simulink model "atakanproje2020a"  (R2020a)
settings: Solver=VariableStepAuto  StartTime=0.0  StopTime=5  RelTol=1e-3
libraries: powerlib x11, powerlib_meascontrol x6, simulink x4, eeAsmScalarControl x1
settings Model: Creator=Atakan  LastModifiedBy=Atakan
settings DebuggingCC: ArithmeticOperatorsInVariantConditions=warning
settings SFSimCC: CustomCodeUndefinedFunction=UseInterfaceOnly

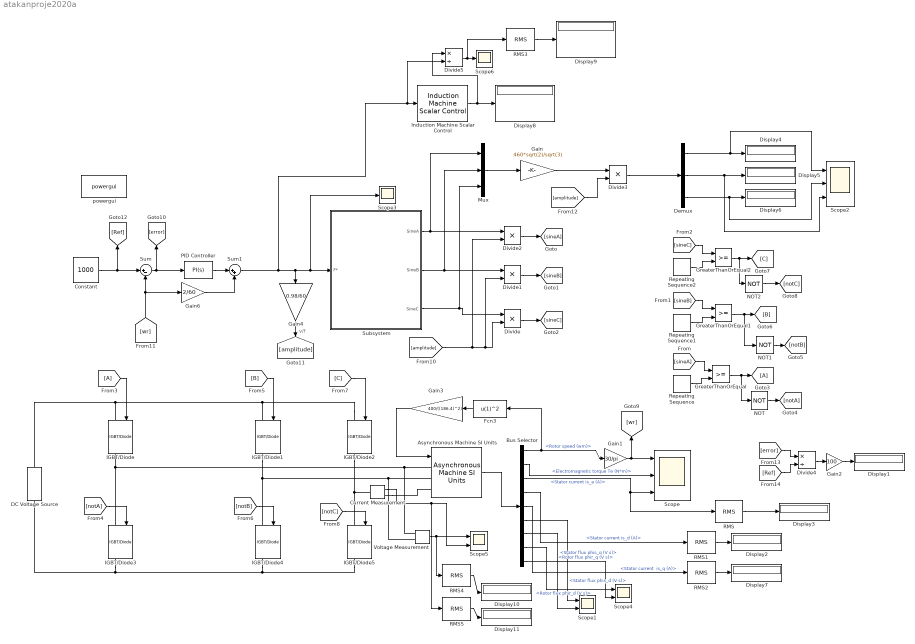
== system atakanproje2020a ==
  note: v/f
  Asynchronous Machine SI Units : powerlib/Machines/Asynchronous Machine SI Units  RotorType=Squirrel-cage  PresetModel="05:  100 HP 460 V 60Hz 1780 RPM"  MechanicalLoad=Torque Tm  ShowDetailedParameters=on  ReferenceFrame=Rotor  Units=SI  MeasurementBus=off  NominalParameters=[7.46e+04 460 60]  Stator=[0.03957 0.000389]  Rotor=[0.02215 0.000389]  Cage1=[0.4155 0.002066]  Cage2=[0.4168 0.0003495]  Lm=0.01664  Mechanical=[1.3 0.05543 2]  PolePairs=2  InitialConditions=[1 0 0 0 0 0 0 0]  SimulateSaturation=off  Saturation=[14.03593122, 27.81365428, 53.79336849, 72.68890987, 97.98006896, 148.6815601, 215.7428561, 302.9841135, 428.7778367 ; 230, 322, 414, 460, 506, 552, 598, 644, 690]  LoadFlowParameters=1492000  TsPowergui=0  TsBlock=-1  IterativeModel=Trapezoidal non iterative  IterativeDiscreteModel=Trapezoidal non iterative  Pmec=1.492e+006
  Bus Selector : BusSelector  OutputSignals="Mechanical.Rotor speed (wm),Mechanical.Electromagnetic torque Te (N*m),Stator measurements.Stator current is_a (A),Stator measurements.Stator current is_d (A),Stator measurements.Stator current  is_q (A),Stator measurements.Stator flux phis_d (V s),Stator measurements.Stator flux phis_q (V s),Rotor measurements.Rotor flux phir_d (V s),Rotor measurements.Rotor flux phir_q (V s)"
  Constant : Constant  Value=1000
  Current Measurement : powerlib/Measurements/Current Measurement  PhasorSimulation=off  OutputType=Complex  PSBequivalent=0
  DC Voltage Source : powerlib/Electrical Sources/DC Voltage Source  Amplitude=800  Measurements=None
  Demux : Demux  Outputs=3
  Display{1..11} (11 alike) : Display
  Divide{,1..3} (4 alike) : Product  Inputs=**
  Divide4 : Product  Inputs=*/
  Divide5 : Product  Inputs=*/
  Fcn3 : Fcn  Expr=u(1)^2
  Gain : Gain  Gain=460*sqrt(2)/sqrt(3)
  Gain1 : Gain  Gain=30/pi
  Gain2 : Gain  Gain=100
  Gain3 : Gain  Gain=400/((186.4)^2)
  Gain4 : Gain  Gain=0.98/60
  Gain6 : Gain  Gain=2/60
  GreaterThanOrEqual : RelationalOperator  OutDataTypeStr=boolean  RndMeth=Simplest
  GreaterThanOrEqual1 : RelationalOperator  OutDataTypeStr=boolean  RndMeth=Simplest
  GreaterThanOrEqual2 : RelationalOperator  OutDataTypeStr=boolean  RndMeth=Simplest
  IGBT/Diode{,1..5} (6 alike) : powerlib/Power Electronics/IGBT//Diode  Ron=1e-3  Rs=1e5  Cs=inf  Measurements=on
  Induction Machine Scalar Control : eeAsmScalarControl/Induction Machine Scalar Control  fn=60  Vn=460  Vmin=10  Ts=-1
      settings: SourceProductBaseCode=PS
  Mux : Mux  Inputs=3
  NOT : Logic  Operator=NOT  AllPortsSameDT=off  OutDataTypeStr=boolean
  NOT1 : Logic  Operator=NOT  AllPortsSameDT=off  OutDataTypeStr=boolean
  NOT2 : Logic  Operator=NOT  AllPortsSameDT=off  OutDataTypeStr=boolean
  PID Controller : simulink/Continuous/PID Controller  Controller=PI  Form=Parallel  TimeDomain=Continuous-time  UseExternalTs=off  SampleTime=-1  IntegratorMethod=Forward Euler  FilterMethod=Forward Euler  ControllerParametersSource=internal  P=0.01  I=0.0001  D=0.000001  UseFilter=on  N=100  TunerSelectOption=Transfer Function Based (PID Tuner App)  InitialConditionSource=internal  InitialConditionForIntegrator=0  InitialConditionForFilter=0  DifferentiatorICPrevScaledInput=0  ExternalReset=none  TrackingMode=off  Kt=1  LimitOutput=on  UpperSaturationLimit=100  LowerSaturationLimit=-100  LinearizeAsGain=on  AntiWindupMode=clamping  Kb=1  POutMin=[]  POutMax=[]  IOutMin=[]  IOutMax=[]  DOutMin=[]  DOutMax=[]  NOutMin=[]  NOutMax=[]  SumOutMin=[]  SumOutMax=[]  SaturationOutMin=[]  SaturationOutMax=[]  PParamMin=[]  PParamMax=[]  IParamMin=[]  IParamMax=[]  DParamMin=[]  DParamMax=[]  NParamMin=[]  NParamMax=[]  KbParamMin=[]  KbParamMax=[]  KtParamMin=[]  KtParamMax=[]  KbOutMin=[]  KbOutMax=[]  KtOutMin=[]  KtOutMax=[]  IntegratorOutMin=[]  IntegratorOutMax=[]  FilterOutMin=[]  FilterOutMax=[]  SumI1OutMin=[]  SumI1OutMax=[]  SumI2OutMin=[]  SumI2OutMax=[]  SumI3OutMin=[]  SumI3OutMax=[]  SumI4OutMin=[]  SumI4OutMax=[]  SumDOutMin=[]  SumDOutMax=[]  DifferentiatorOutMin=[]  DifferentiatorOutMax=[]  FilterDiffOutCoefMin=[]  FilterDiffOutCoefMax=[]  ReciprocalOutMin=[]  ReciprocalOutMax=[]  SumDenOutMin=[]  SumDenOutMax=[]  SumNumOutMin=[]  SumNumOutMax=[]  DivideOutMin=[]  DivideOutMax=[]  UdiffTsProdOutMin=[]  UdiffTsProdOutMax=[]  NTsProdOutMin=[]  NTsProdOutMax=[]  UintegralTsProdOutMin=[]  UintegralTsProdOutMax=[]  UngainTsProdOutMin=[]  UngainTsProdOutMax=[]  IntegratorContinuousStateAttributes=''  IntegratorStateMustResolveToSignalObject=off  IntegratorRTWStateStorageClass=Auto  FilterContinuousStateAttributes=''  FilterStateMustResolveToSignalObject=off  FilterRTWStateStorageClass=Auto  ParallelPVariant=InternalParameters  IdealPVariant=Disabled  IVariant=InternalParameters  DVariant=Disabled  IntegratorVariant=Continuous  SatVariant=Enabled  AWVariant=ContClampingParallel  PCopyVariant=Disabled  TRVariant=Disabled  FdbkBlocksVariant=Forward  IdealPFdbkVariant=Disabled  SatFdbkVariant=Disabled  DerivativeFilterVariant=Disabled  NVariant=Disabled  NCopyVariant=Disabled_SignalSpec  FilterICVariant=Disabled  IntegratorICVariant=InternalICs  ExternalResetVariant=Disabled  TRSumVariant=Passthrough  SumFdbkVariant=Disabled  SumVariant=Sum_PI  TsampFilterVariant=InternalTs  TsampNgainVariant=Passthrough  TsampIntegralVariant=Passthrough
  RMS{,1..5} (6 alike) : powerlib_meascontrol/Measurements/RMS  TrueRMS=on  Freq=60  RMSInit=120  Ts=0
  Repeating Sequence : simulink/Sources/Repeating Sequence  rep_seq_t=[0 0.25 0.5 0.75 1]/2000  rep_seq_y=[0 1 0 -1 0]
  Repeating Sequence1 : simulink/Sources/Repeating Sequence  rep_seq_t=[0 0.25 0.5 0.75 1]/2000  rep_seq_y=[0 1 0 -1 0]
  Repeating Sequence2 : simulink/Sources/Repeating Sequence  rep_seq_t=[0 0.25 0.5 0.75 1]/2000  rep_seq_y=[0 1 0 -1 0]
  Scope : Scope  NumInputPorts=3
  Scope1 : Scope  NumInputPorts=2
  Scope2 : Scope  NumInputPorts=3
  Scope3 : Scope
  Scope4 : Scope  NumInputPorts=2
  Scope5 : Scope  NumInputPorts=2
  Scope6 : Scope
  Subsystem : Subsystem
  Sum : Sum  Inputs=|+-
  Sum1 : Sum  Inputs=|++
  Voltage Measurement : powerlib/Measurements/Voltage Measurement  PhasorSimulation=off  OutputType=Complex  PSBequivalent=0
  powergui : powerlib/powergui  Priority=1  SimulationMode=Discrete  SampleTime=50e-6  frequency=60  Iterations=50  frequencyindice=60  Pbase=100e6  ErrMax=1e-4  UnitsV=kV  UnitsW=MW  buscounter=0  FunctionMessages=off  echomessages=off  EnableUseOfTLC=off  CurrentSourceSwitches=off  DisableSnubberDevices=off  DisableRonSwitches=off  DisableVfSwitches=off  DisplayEquations=off  AutomaticDiscreteSolvers=off  SolverType=Tustin/Backward Euler (TBE)  Interpol=off  ExternalGateDelay=off  methode=off  Ts=100  x0status=blocks  SPID=on  SwTol=0  HookPort=off  NonlinearTolerance=1e-4  nMaxIteration=100  ContinueOnMaxIteration=off  RestoreLinks=warning  ResistiveCurrentMeasurement=off  Frange=[0:2:500]  Ylog=off  Xlog=on  ShowGrid=off  save=off  variable=ZData  structure=0  ZoomFFT=off  StartTime=0.0  cycles=1  DisplayStyle=1  fundamental=60  FreqAxis=off  MaxFrequency=1000  frequencyindicesteady=1  RmsSteady=1  display=off
  wires:
  Sum/1 -> PID Controller/1, [error]
  Repeating Sequence/1 -> GreaterThanOrEqual/2
  [sineA] -> GreaterThanOrEqual/1
  Repeating Sequence1/1 -> GreaterThanOrEqual1/2
  [sineB] -> GreaterThanOrEqual1/1
  Repeating Sequence2/1 -> GreaterThanOrEqual2/2
  [sineC] -> GreaterThanOrEqual2/1
  GreaterThanOrEqual/1 -> NOT/1, [A]
  NOT/1 -> [notA]
  NOT1/1 -> [notB]
  GreaterThanOrEqual1/1 -> NOT1/1, [B]
  NOT2/1 -> [notC]
  GreaterThanOrEqual2/1 -> NOT2/1, [C]
  [A] -> IGBT/Diode/1
  [notA] -> IGBT/Diode3/1
  [B] -> IGBT/Diode1/1
  [notB] -> IGBT/Diode4/1
  [C] -> IGBT/Diode2/1
  [notC] -> IGBT/Diode5/1
  Asynchronous Machine SI Units/1 -> Bus Selector/1
  Bus Selector/1 -> Gain1/1, Fcn3/1  "<Rotor speed (wm)>"
  Bus Selector/2 -> Scope/2  "<Electromagnetic torque Te (N*m)>"
  Fcn3/1 -> Gain3/1
  Gain3/1 -> Asynchronous Machine SI Units/1
  Gain1/1 -> [wr], Scope/1
  Constant/1 -> [Ref], Sum/1
  [amplitude] -> Divide2/2, Divide1/2, Divide/2
  Subsystem/3(SineC) -> Mux/3, Divide/1
  Divide/1 -> [sineC]
  Subsystem/2(SineB) -> Mux/2, Divide1/1
  Subsystem/1(SineA) -> Mux/1, Divide2/1
  Divide2/1 -> [sineA]
  Divide1/1 -> [sineB]
  Gain4/1 -> [amplitude]
  [wr] -> Gain6/1, Sum/2
  Bus Selector/3 -> RMS/1, Scope/3  "<Stator current is_a (A)>"
  PID Controller/1 -> Sum1/1
  Gain6/1 -> Sum1/2
  Sum1/1 -> Divide5/2, Induction Machine Scalar Control/1, Scope3/1, Subsystem/1(F*), Gain4/1
  Mux/1 -> Gain/1
  Gain/1 -> Divide3/1
  [amplitude] -> Divide3/2
  Divide3/1 -> Demux/1
  Demux/3 -> Scope2/2, Display6/1
  Demux/1 -> Scope2/1, Display4/1
  Bus Selector/4 -> RMS1/1  "<Stator current is_d (A)>"
  Bus Selector/5 -> RMS2/1  "<Stator current  is_q (A)>"
  RMS/1 -> Display3/1
  [Ref] -> Divide4/2
  [error] -> Divide4/1
  Divide4/1 -> Gain2/1
  Gain2/1 -> Display1/1
  Demux/2 -> Scope2/3, Display5/1
  RMS2/1 -> Display7/1
  RMS1/1 -> Display2/1
  Bus Selector/6 -> Scope1/1  "<Stator flux phis_d (V s)>"
  Bus Selector/7 -> Scope1/2  "<Stator flux phis_q (V s)>"
  Bus Selector/8 -> Scope4/1  "<Rotor flux phir_d (V s)>"
  Bus Selector/9 -> Scope4/2  "<Rotor flux phir_q (V s)>"
  Induction Machine Scalar Control/1 -> Divide5/1, Display8/1
  Divide5/1 -> RMS3/1, Scope6/1
  RMS3/1 -> Display9/1
  Voltage Measurement/1 -> RMS4/1, Scope5/1
  Current Measurement/1 -> RMS5/1, Scope5/2
  RMS4/1 -> Display10/1
  RMS5/1 -> Display11/1
  connections:
  DC Voltage Source/LConn1 -- IGBT/Diode5/RConn1 -- IGBT/Diode4/RConn1 -- IGBT/Diode3/RConn1
  IGBT/Diode2/LConn1 -- DC Voltage Source/RConn1 -- IGBT/Diode/LConn1 -- IGBT/Diode1/LConn1
  IGBT/Diode3/LConn1 -- Voltage Measurement/LConn1 -- Asynchronous Machine SI Units/LConn1 -- IGBT/Diode/RConn1
  IGBT/Diode2/RConn1 -- Current Measurement/LConn1 -- IGBT/Diode5/LConn1
  IGBT/Diode1/RConn1 -- Voltage Measurement/LConn2 -- Asynchronous Machine SI Units/LConn2 -- IGBT/Diode4/LConn1
  Current Measurement/RConn1 -- Asynchronous Machine SI Units/LConn3

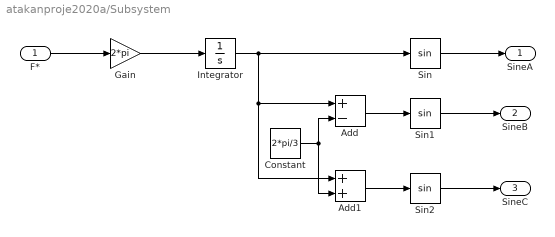
== system atakanproje2020a/Subsystem ==
  F* : Inport
  Add : Sum  Inputs=+-
  Add1 : Sum
  Constant : Constant  Value=2*pi/3
  Gain : Gain  Gain=2*pi
  Integrator : Integrator
  Sin : Trigonometry
  Sin1 : Trigonometry
  Sin2 : Trigonometry
  SineA : Outport
  SineB : Outport  Port=2
  SineC : Outport  Port=3
  wires:
  Add/1 -> Sin1/1
  Sin/1 -> SineA/1
  Sin1/1 -> SineB/1
  Sin2/1 -> SineC/1
  Constant/1 -> Add1/2, Add/2
  Integrator/1 -> Sin/1, Add/1, Add1/1
  F*/1 -> Gain/1
  Add1/1 -> Sin2/1
  Gain/1 -> Integrator/1
